simulink model "circuit5diskr"  (Simulink 5.0)
settings: Solver=ode1  StartTime=0.0  StopTime=1  FixedStep=10e-6  RelTol=1e-4
libraries: powerlib2 x10, powerlib_extras x3
settings Model: LastModifiedBy=Администратор

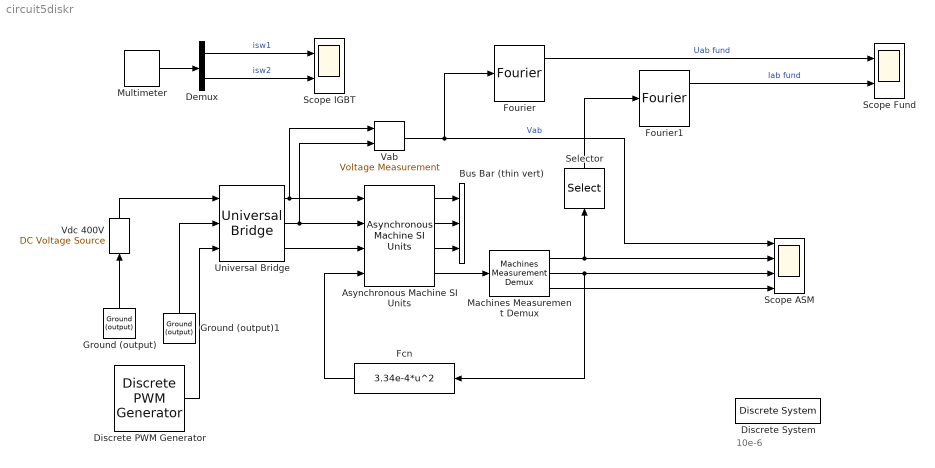
== system circuit5diskr ==
  note: 10e-6
  Asynchronous Machine SI Units : powerlib2/Machines/Asynchronous Machine SI Units  Tag=PoWeRsYsTeMbLoCk  rotType=Wound  ctrl=Rotor  x1=[ 3*746, 220, 60 ]  x2="[ 0.435  2.0e-3 ]"  x3="[ 0.816  2.0e-3 ]"  x4=69.31e-3  x5="[ 0.089  0  2 ]"  x6="[ 1,0   0,0,0   0,0,0 ]"  PSBOutputType=1110  iounits=1  LoadFlowParameters=0
  Bus Bar (thin vert) : powerlib2/Connectors/Bus Bar (thin vert)  Tag=PoWeRsYsTeMbLoCk  input=3  output=0  PSBOutputType=111111111111111111111111111111111111111111111111111111111111111111111111111111111111
  Demux : Demux  Outputs=2
  Discrete PWM Generator : powerlib_extras/Discrete  Control Blocks/Discrete PWM Generator  GeneratorMode="3-arm  bridge (6 pulses)"  Fc=1080  Ts=10e-6  Internal=on  mIndex=0.9  Freq=60  Phase=0
  Discrete System : powerlib2/Discrete System  methode=0  Ts=10e-6
  Fcn : Fcn  Orientation=left  Expr=3.34e-4*u^2
  Fourier : powerlib_extras/Measurements/Fourier  f1=60  n=1
  Fourier1 : powerlib_extras/Measurements/Fourier  f1=60  n=1
  Ground (output) : powerlib2/Connectors/Ground (output)  Tag=PoWeRsYsTeMbLoCk  Orientation=up  PSBOutputType=1
  Ground (output)1 : powerlib2/Connectors/Ground (output)  Tag=PoWeRsYsTeMbLoCk  Orientation=up  PSBOutputType=1
  Machines Measurement Demux : powerlib2/Machines/Machines Measurement Demux  machType=Asynchronous  ssm1=on  ssm2=on  ssm3=on  ssm4=on  ssm5=on  ssm6=on  sm1=on  sm2=off  sm3=off  sm4=off  sm5=off  sm6=off  sm7=off  sm8=on  sm9=off  sm10=off  sm11=off  sm115=on  sm12=off  sm13=off  sm14=off  asm1=off  asm2=off  asm3=off  asm4=off  asm5=on  asm6=off  asm7=off  asm8=off  asm9=on  asm10=on  asm11=off  pmsm1=on  pmsm2=on  pmsm3=on  pmsm4=on  pmsm5=on  pmsm6=on  lastType=1
  Multimeter : powerlib2/Measurements/Multimeter  Tag=PoWeRsYsTeMmEaSuReMeNt  PhasorSimulation=off  OutputType=Magnitude  sel=[1 2]  L=6  Gain=[1 1]  yselected={'Isw1: Universal Bridge','Isw2: Universal Bridge'};  PSBOutputType=1  PSBequivalent=0  AxesSetting=[0,0.1,-100,100]  Display=1  SavedBlockNames=-11
  Scope ASM : Scope  NumInputPorts=4
      settings: YMin=-500~-75~97.5~42.5  YMax=500~75~122.5~57.5
  Scope Fund : Scope  NumInputPorts=2
      settings: YMin=275~78  YMax=292.5~83
  Scope IGBT : Scope  NumInputPorts=2
      settings: YMin=275~78  YMax=292.5~83  SaveName=ScopeData2
  Selector : Selector  Orientation=up  InputPortWidth=3
  Universal Bridge : powerlib2/Power Electronics/Universal Bridge  Tag=PoWeRsYsTeMbLoCk  arms=3  confi=ABC as output terminals  injcc=1e5  cf=inf  device=IGBT / Diodes  Ron=1e-3  Lon=0  VFs="[  0  0  ]"  Vf=0  gtoparameters=[ 10e-6 , 20e-6 ]  igbtparameters=[ 1e-6 , 1e-6 ]  mesure=Device currents  PSBOutputType=111
  Vab : powerlib2/Measurements/Voltage Measurement  Tag=PoWeRsYsTeMmEaSuReMeNt  PhasorSimulation=off  OutputType=Magnitude  PSBOutputType=0  PSBequivalent=1
  Vdc 400V : powerlib2/Electrical Sources/DC Voltage Source  Tag=PoWeRsYsTeMbLoCk  Description=source block  Orientation=up  V=400  mesure=None  PSBOutputType=1
  wires:
  Universal Bridge/1 -> Asynchronous Machine SI Units/1, Vab/1
  Universal Bridge/2 -> Asynchronous Machine SI Units/2, Vab/2
  Universal Bridge/3 -> Asynchronous Machine SI Units/3
  Asynchronous Machine SI Units/1 -> Bus Bar (thin vert)/1
  Asynchronous Machine SI Units/2 -> Bus Bar (thin vert)/2
  Asynchronous Machine SI Units/3 -> Bus Bar (thin vert)/3
  Asynchronous Machine SI Units/4 -> Machines Measurement Demux/1
  Machines Measurement Demux/2 -> Fcn/1, Scope ASM/3
  Fcn/1 -> Asynchronous Machine SI Units/4
  Vdc 400V/1 -> Universal Bridge/1
  Ground (output)/1 -> Vdc 400V/1
  Ground (output)1/1 -> Universal Bridge/2
  Discrete PWM Generator/1 -> Universal Bridge/3
  Vab/1 -> Fourier/1, Scope ASM/1  "Vab"
  Machines Measurement Demux/1 -> Selector/1, Scope ASM/2
  Selector/1 -> Fourier1/1
  Fourier/1 -> Scope Fund/1  "Uab fund"
  Fourier1/1 -> Scope Fund/2  "Iab fund"
  Machines Measurement Demux/3 -> Scope ASM/4
  Multimeter/1 -> Demux/1
  Demux/1 -> Scope IGBT/1  "isw1"
  Demux/2 -> Scope IGBT/2  "isw2"
